simulink model "swps_2_xfer"  (Simulink 7.0)
settings: Solver=ode23s  StartTime=0.0  StopTime=inf  MaxStep=.02/50e3  RelTol=1e-3
values from neighbouring files (symbols this model uses):
  a = [1 5726094.8537 1.28575913301e+14 5.9794238322e+20 5.92198785204e+27 2.12389820757e+34 1.13681638083e+41 2.81062253129e+47 7.3943533776e+53 8.72896491872e+59]    [lpf_coefs.mat]
  b = [0 36927.0233589 -2.57790101622e-05 1.2013848239e+19 -1092387632.02 1.28157428918e+33 2.40587360249e+23 5.61084731217e+46 9.8548958414e+36 8.72896491872e+59]    [lpf_coefs.mat]
undefined symbols (not defined in the file or in its folder): c, d, dfilt, gcbh, magnitude, powericon
libraries: powerlib x9, dspindex x8, dspsigops x4, dspbuff3 x3, dspxfrm3 x3, dsparch4 x2, dspsnks4 x2, dspsrcs4 x1, dspmtrx3 x1, simulink x1, simulink_extras x1
CloseFcn:
  | rtwprivate ssgencode ModelCloseRequest swps_2
settings Model: Creator=dbenson  LastModifiedBy=Owner
settings SolverCC: InitialStep=.01/50e3  ZeroCrossControl=EnableAll
settings DataIOCC: LimitDataPoints=off  SaveOutput=off  SignalLogging=off  SaveTime=off  SignalLoggingName=sigsOut
settings OptimizationCC: BooleanDataType=off  OptimizeModelRefInitCode=on  LifeSpan=1
settings DebuggingCC: SaveWithParameterizedLinksMsg=none  SignalResolutionControl=TryResolveAllWithWarning  SolverPrmCheckMsg=none  MultiTaskDSMMsg=warning  MultiTaskCondExecSysMsg=none  StrictBusMsg=None
settings RTWCC: SystemTargetFile=ert.tlc  TemplateMakefile=ert_default_tmf  Description=Real-Time Workshop Embedded Coder (no auto configuration)  GenerateReport=on  ProcessScript=ert_make_rtw_hook  IncludeHyperlinkInReport=on  LaunchReport=on  IncludeERTFirstTime=on
settings CodeAppCC: IgnoreCustomStorageClasses=off
settings ERTTargetCC: TargetFcnLib=ansi_tfl_tmw.mat  GenFloatMathFcnCalls=ANSI_C  GenerateSampleERTMain=on  GenerateErtSFunction=on  InlinedParameterPlacement=NonHierarchical  ERTCustomFileTemplate=example_file_process.tlc

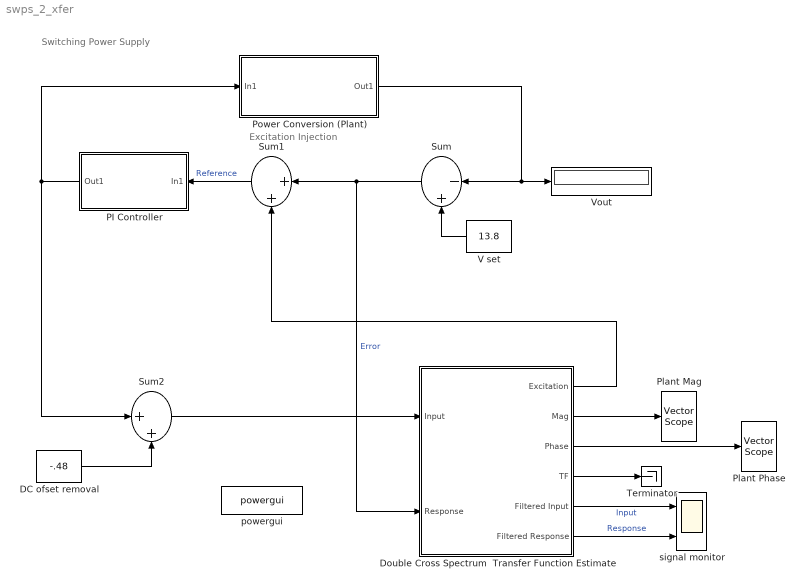
== system swps_2_xfer ==
  note: Switching Power Supply
  note: Excitation Injection
  DC ofset removal : Constant  Value=-.48  OutDataType=sfix(16)  OutScaling=2^0
  Double Cross Spectrum  Transfer Function Estimate : Subsystem  Description=Spectrum Analyzer  mask{BW=5e3, NFFT=128, Level=.02, Chirp=off, Avg_fac=10, Nholdoff=2, Unwrap=off}
      mask prompts: BW "Bandwidth (Hz)"; NFFT "FFT Length (power of 2)"; Level "Excitation Level"; Chirp "Chirp Excitation"; Avg_fac "Averaging Factor (>=1)"; Nholdoff "Hold Off  (in Frames)"; Unwrap "Unwrap Phase"
  PI Controller : Subsystem  Orientation=left
  Plant Mag : dspsnks4/Vector Scope  DialogController=dspdialog.VectorScope  DialogControllerArgs=DataTag9  ScopeProperties=on  Domain=Frequency  HorizSpan=1  DisplayProperties=off  AxisGrid=on  Memory=off  FrameNumber=on  AxisLegend=off  AxisZoom=off  OpenScopeAtSimStart=on  OpenScopeImmediately=off  FigPos=[7 35 334 255]  AxisProperties=off  XUnits=Hertz  XRange=[0...Fs/2]  InheritXIncr=on  XIncr=1  XLabel=Time  XLimit=Auto  XMin=0  XMax=1  XStart=0  YUnits=dB  YLabel=Amplitude  LineProperties=off
      settings: YMin=-30  YMax=30
  Plant Phase : dspsnks4/Vector Scope  DialogController=dspdialog.VectorScope  DialogControllerArgs=DataTag10  ScopeProperties=on  Domain=Frequency  HorizSpan=1  DisplayProperties=off  AxisGrid=on  Memory=off  FrameNumber=on  AxisLegend=off  AxisZoom=off  OpenScopeAtSimStart=on  OpenScopeImmediately=off  FigPos=[350 28 337 266]  AxisProperties=off  XUnits=Hertz  XRange=[0...Fs/2]  InheritXIncr=on  XIncr=1  XLabel=Time  XLimit=Auto  XMin=0  XMax=1  XStart=0  YUnits=Magnitude  YLabel=Phase  LineProperties=off
      settings: YMin=-50  YMax=200
  Power Conversion (Plant) : Subsystem
  Sum : Sum  Orientation=left  Inputs=|-+  OutDataType=sfix(16)  OutScaling=2^0  SaturateOnIntegerOverflow=on  InputSameDT=on
  Sum1 : Sum  Orientation=left  Inputs=|++  OutDataType=sfix(16)  OutScaling=2^0  SaturateOnIntegerOverflow=on  InputSameDT=on
  Sum2 : Sum  Inputs=|++  OutDataType=sfix(16)  OutScaling=2^0  SaturateOnIntegerOverflow=on  InputSameDT=on
  Terminator : Terminator
  "V set " : Constant  Orientation=left  Value=13.8  OutDataType=sfix(16)  OutScaling=2^0
  Vout : Display
      settings: Decimation=20
  powergui : powerlib/powergui  SystemSampleTime=-1  SimulationMode=Continuous  SampleTime=0  echomessages=off  RestoreLinks=warning  x0status=blocks  Frange=[0:2:500]  Ylog=off  Xlog=on  ShowGrid=off  save=off  variable=ZData  ZoomFFT=on  StartTime=0.0  cycles=1  DisplayStyle=1  fundamental=60  FreqAxis=off  MaxFrequency=1000  frequencyindice=0  frequencyindicesteady=1  RmsSteady=1  display=off  Ts=0  frequency=60  methode=off  HookPort=off  Interpol=off  SPID=off  FunctionMessages=off
  signal monitor : Scope  NumInputPorts=2
      settings: TimeRange=0.01  YMin=-0.75~-0.3  YMax=0.75~0.25  SaveName=ScopeData2
  wires:
  "V set "/1 -> Sum/2
  Power Conversion (Plant)/1(Out1) -> Sum/1, Vout/1
  PI Controller/1(Out1) -> Power Conversion (Plant)/1(In1), Sum2/1
  Sum/1 -> Sum1/1, Double Cross Spectrum  Transfer Function Estimate/2(Response)  "Error"
  Sum1/1 -> PI Controller/1(In1)  "Reference"
  Double Cross Spectrum  Transfer Function Estimate/2(Mag) -> Plant Mag/1
  Double Cross Spectrum  Transfer Function Estimate/3(Phase) -> Plant Phase/1
  Double Cross Spectrum  Transfer Function Estimate/1(Excitation) -> Sum1/2
  DC ofset removal/1 -> Sum2/2
  Double Cross Spectrum  Transfer Function Estimate/4(TF) -> Terminator/1
  Sum2/1 -> Double Cross Spectrum  Transfer Function Estimate/1(Input)
  Double Cross Spectrum  Transfer Function Estimate/5(Filtered Input) -> signal monitor/1  "Input"
  Double Cross Spectrum  Transfer Function Estimate/6(Filtered Response) -> signal monitor/2  "Response"

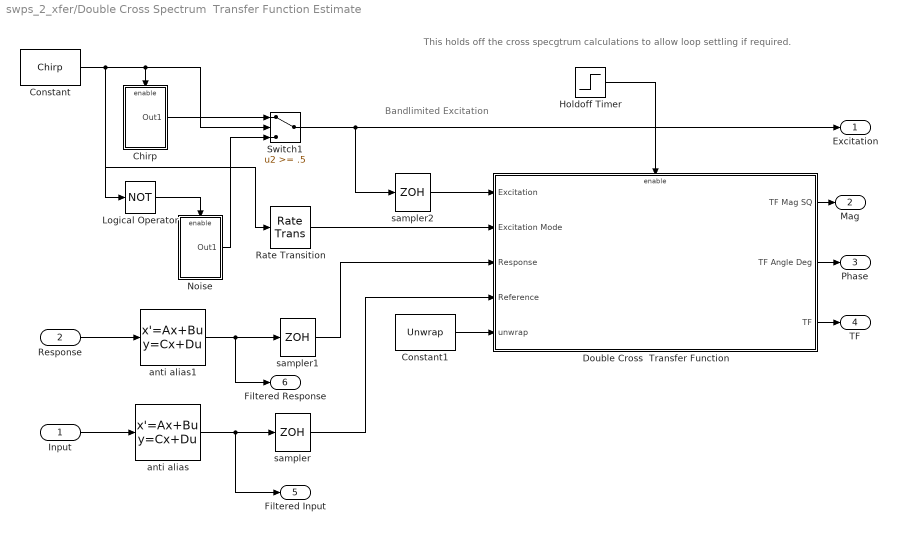
== system swps_2_xfer/Double Cross Spectrum  Transfer Function Estimate ==
  note: This holds off the cross specgtrum calculations
      |  to allow loop settling if required.
  note: Bandlimited Excitation
  Input : Inport  OutDataType=sfix(16)  OutScaling=2^0
  Response : Inport  Port=2  OutDataType=sfix(16)  OutScaling=2^0
  Chirp : Subsystem
  Constant : Constant  Value=Chirp  OutDataType=sfix(16)  OutScaling=2^0
  Constant1 : Constant  Value=Unwrap  OutDataType=sfix(16)  OutScaling=2^0
  "Double Cross  Transfer Function " : Subsystem  mask{NFFT=NFFT, Navg=Avg_fac, pcnt=100/1.28, BW=BW}
      mask prompts: NFFT "FFT length (power of 2):"; Navg "Spectral Averaging Factor (>=1):"; pcnt "Percentage of  Alias Free Data  (<=100)"; BW "Bandwidth"
      mask Display: disp('Double Cross\n Transfer Function \n Estimation (v1.0) ')
  Holdoff Timer : Step  Time=Nholdoff*NFFT/(2.56*BW)  SampleTime=1/(2.56*BW)
  Logical Operator : Logic  Operator=NOT  AllPortsSameDT=off  OutDataTypeMode=boolean
  Noise : Subsystem
  Rate Transition : RateTransition
  Switch1 : Switch  Threshold=.5
  anti alias : StateSpace  AncestorBlock=dsparch3/Analog Filter Design  A=a  B=b  C=c  D=d  mask(Analog Filter Design){method=Elliptic, filttype=Lowpass, N=8, Wlo=BW*2*pi, Whi=80, Rp=2, Rs=100}
      mask prompts: method "Design method:"; filttype "Filter type:"; N "Filter order:"; Wlo "Passband edge frequency (rad/s):"; Whi "(unused)"; Rp "Passband ripple in dB:"; Rs "Stopband attenuation in dB:"
      mask help: Design one of several standard analog filters, implemented in state-space form.
      mask init:
      | [a,b,c,d,h,w,str]=dspblkanalog('design', method,filttype,N,Wlo,Whi,Rp,Rs);
      mask Help: web(dspbhelp);
      mask StyleString: popup(Butterworth|Chebyshev I|Chebyshev II|Elliptic|Bessel),popup(Lowpass|Highpass|Bandpass|Bandstop),edit,edit,edit,edit,edit
      mask CallbackString: dspblkanalog|dspblkanalog|||||
      mask Display: plot(w,h); text(.05,.9,str);
  anti alias1 : StateSpace  AncestorBlock=dsparch3/Analog Filter Design  A=a  B=b  C=c  D=d  mask(Analog Filter Design){method=Elliptic, filttype=Lowpass, N=8, Wlo=BW*2*pi, Whi=80, Rp=2, Rs=100}
      mask prompts: method "Design method:"; filttype "Filter type:"; N "Filter order:"; Wlo "Passband edge frequency (rad/s):"; Whi "(unused)"; Rp "Passband ripple in dB:"; Rs "Stopband attenuation in dB:"
      mask help: Design one of several standard analog filters, implemented in state-space form.
      mask init:
      | [a,b,c,d,h,w,str]=dspblkanalog('design', method,filttype,N,Wlo,Whi,Rp,Rs);
      mask Help: web(dspbhelp);
      mask StyleString: popup(Butterworth|Chebyshev I|Chebyshev II|Elliptic|Bessel),popup(Lowpass|Highpass|Bandpass|Bandstop),edit,edit,edit,edit,edit
      mask CallbackString: dspblkanalog|dspblkanalog|||||
      mask Display: plot(w,h); text(.05,.9,str);
  sampler : ZeroOrderHold  SampleTime=1/(2.56*BW)
  sampler1 : ZeroOrderHold  SampleTime=1/(2.56*BW)
  sampler2 : ZeroOrderHold  SampleTime=1/(2.56*BW)
  Excitation : Outport  OutDataType=sfix(16)  OutScaling=2^0
  Mag : Outport  Port=2  OutDataType=sfix(16)  OutScaling=2^0
  Phase : Outport  Port=3  OutDataType=sfix(16)  OutScaling=2^0
  TF : Outport  Port=4  OutDataType=sfix(16)  OutScaling=2^0
  Filtered Input : Outport  Port=5  OutDataType=sfix(16)  OutScaling=2^0
  Filtered Response : Outport  Port=6  OutDataType=sfix(16)  OutScaling=2^0
  wires:
  "Double Cross  Transfer Function "/3("TF ") -> TF/1
  sampler/1 -> "Double Cross  Transfer Function "/4(Reference)
  "Double Cross  Transfer Function "/1(TF Mag SQ) -> Mag/1
  "Double Cross  Transfer Function "/2(TF Angle Deg) -> Phase/1
  Holdoff Timer/1 -> "Double Cross  Transfer Function "/Enable
  anti alias/1 -> Filtered Input/1, sampler/1
  Input/1 -> anti alias/1
  anti alias1/1 -> sampler1/1, Filtered Response/1
  Response/1 -> anti alias1/1
  sampler1/1 -> "Double Cross  Transfer Function "/3(Response)
  Chirp/1(Out1) -> Switch1/1
  Noise/1(Out1) -> Switch1/3
  Switch1/1 -> Excitation/1, sampler2/1
  Constant/1 -> Logical Operator/1, Chirp/Enable, Switch1/2, Rate Transition/1
  Logical Operator/1 -> Noise/Enable
  Constant1/1 -> "Double Cross  Transfer Function "/5(unwrap)
  sampler2/1 -> "Double Cross  Transfer Function "/1(Excitation)
  Rate Transition/1 -> "Double Cross  Transfer Function "/2(Excitation Mode)

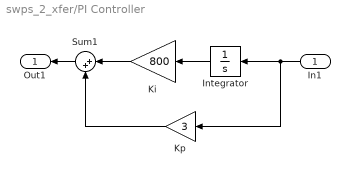
== system swps_2_xfer/PI Controller ==
  In1 : Inport  Orientation=left
  Integrator : Integrator  Orientation=left
  Ki : Gain  Orientation=left  Gain=800  ParameterDataType=sfix(16)  ParameterScaling=2^0  OutDataType=sfix(16)  OutScaling=2^0
  Kp : Gain  Orientation=left  Gain=3  ParameterDataType=sfix(16)  ParameterScaling=2^0  OutDataType=sfix(16)  OutScaling=2^0
  Sum1 : Sum  Orientation=left  Inputs=|++  OutDataType=sfix(16)  OutScaling=2^0  SaturateOnIntegerOverflow=on  InputSameDT=on
  Out1 : Outport  Orientation=left
  wires:
  In1/1 -> Kp/1, Integrator/1
  Integrator/1 -> Ki/1
  Kp/1 -> Sum1/2
  Sum1/1 -> Out1/1
  Ki/1 -> Sum1/1

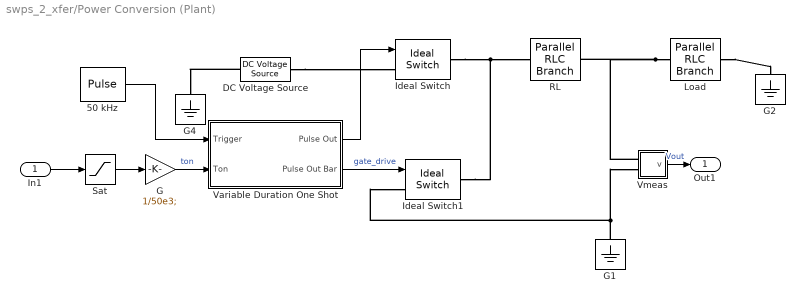
== system swps_2_xfer/Power Conversion (Plant) ==
  In1 : Inport
  50 kHz : DiscretePulseGenerator  PulseType=Time based  Period=1/50e3;  PulseWidth=50  PhaseDelay=1e-6
  DC Voltage Source : powerlib/Electrical Sources/DC Voltage Source  Description=source block  DialogController=POWERSYS.PowerSysDialog  SystemSampleTime=-1  Amplitude=30  Measurements=None
      settings: AttributesFormatString=\n
  G : Gain  Gain=1/50e3;  ParameterDataType=sfix(16)  ParameterScaling=2^0  OutDataType=sfix(16)  OutScaling=2^0  SaturateOnIntegerOverflow=on
  G1 : powerlib/Elements/Ground  Orientation=down  DialogController=POWERSYS.PowerSysDialog  PhysicalDomain=powersysdomain  SubClassName=unknown  LeftPortType=p1  RightPortType=p1  LConnTagsString=a
  G2 : powerlib/Elements/Ground  Orientation=down  DialogController=POWERSYS.PowerSysDialog  PhysicalDomain=powersysdomain  SubClassName=unknown  LeftPortType=p1  RightPortType=p1  LConnTagsString=a
  G4 : powerlib/Elements/Ground  Orientation=down  DialogController=POWERSYS.PowerSysDialog  PhysicalDomain=powersysdomain  SubClassName=unknown  LeftPortType=p1  RightPortType=p1  LConnTagsString=a
  Ideal Switch : powerlib/Power Electronics/Ideal Switch  DialogController=POWERSYS.PowerSysDialog  SystemSampleTime=-1  Ron=0.1  Lon=0  IC=0  Rs=0  Cs=0  Measurements=off
      settings: AttributesFormatString=\n
  Ideal Switch1 : powerlib/Power Electronics/Ideal Switch  DialogController=POWERSYS.PowerSysDialog  SystemSampleTime=-1  Ron=0.1  Lon=0  IC=0  Rs=0  Cs=0  Measurements=off
      settings: AttributesFormatString=\n
  Load : powerlib/Elements/Parallel RLC Branch  DialogController=POWERSYS.PowerSysDialog  PhysicalDomain=powersysdomain  SubClassName=unknown  LeftPortType=p1  RightPortType=p1  LConnTagsString=a  RConnTagsString=__new0  BranchType=RC  Resistance=2  Inductance=1.0  SetiL0=off  InitialCurrent=0  Capacitance=47e-6  Setx0=off  InitialVoltage=13.8  Measurements=None
  RL : powerlib/Elements/Parallel RLC Branch  DialogController=POWERSYS.PowerSysDialog  PhysicalDomain=powersysdomain  SubClassName=unknown  LeftPortType=p1  RightPortType=p1  LConnTagsString=a  RConnTagsString=__new0  BranchType=RL  Resistance=10000  Inductance=1e-3  SetiL0=off  InitialCurrent=0  Capacitance=1.0  Setx0=off  InitialVoltage=0  Measurements=None
  Sat : Saturate  UpperLimit=0.95  LowerLimit=.001
  Variable Duration One Shot : Subsystem
  Vmeas : Subsystem  Tag=PoWeRsYsTeMmEaSuReMeNt  AncestorBlock=powerlib/Measurements/Voltage Measurement  LoadFcn=powericon('psbloadfunction',gcbh,'Measurement Block','');  InitFcn=powericon('psbloadfunction',gcbh,'InitFcnOfSPSBlocks','Measurement Block');  mask(Voltage Measurement){PhasorSimulation=off, OutputType=Magnitude, PSBequivalent=0}
      mask prompts: PhasorSimulation "Phasor simulation"; OutputType "Output signal :"; PSBequivalent "Equivalent circuit"
      mask help: Ideal voltage measurement.
      mask init:
      | switch OutputType
      | case 1
      |     OutputSelection = 1;
      |     NormalMode = 2;
      |     PhasorMode = 1;
      | case 2
      |     OutputSelection =[2,3];
      |     NormalMode = 3;
      |     PhasorMode = [1,2];
      | case 3
      |     OutputSelection =[4,5];
      |     NormalMode = 3;
      |     PhasorMode = [1,2];
      | case 4
      |     OutputSelection =[4];
      |     NormalMode = 2;
      |     PhasorMode = 1;
      | end
      | %
      | if PhasorSimulation
      |     SelectionMode = PhasorMode;
      | else
      |     SelectionMode = NormalMode;
      | end
      settings: AttributesFormatString=\n  CopyFcn=powericon('psbloadfunction',gcbh,'Measurement Block','VerifyPhasor');  PreSaveFcn=powericon('psbloadfunction',gcbh,'ModelCloseFcn','');  CloseFcn=powericon('psbloadfunction',gcbh,'CloseFcn','');
      mask Help: web(psbhelp);
      mask StyleString: checkbox,popup(Complex|Real-Imag|Magnitude-Angle|Magnitude),edit
  Out1 : Outport
  wires:
  50 kHz/1 -> Variable Duration One Shot/1(Trigger)
  G/1 -> Variable Duration One Shot/2(Ton)  "ton"
  Sat/1 -> G/1
  Variable Duration One Shot/1(Pulse Out) -> Ideal Switch/1
  Variable Duration One Shot/2(Pulse Out Bar) -> Ideal Switch1/1  "gate_drive"
  In1/1 -> Sat/1
  Vmeas/1(v) -> Out1/1  "Vout"
  connections:
  DC Voltage Source/LConn1 -- G4/LConn1
  DC Voltage Source/RConn1 -- Ideal Switch/LConn1
  G1/LConn1 -- Vmeas/LConn2 -- Ideal Switch1/LConn1
  Load/RConn1 -- G2/LConn1
  Ideal Switch/RConn1 -- Ideal Switch1/RConn1 -- RL/LConn1
  Load/LConn1 -- RL/RConn1 -- Vmeas/LConn1

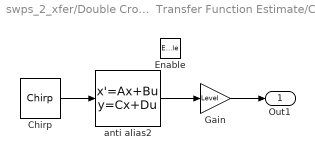
== system swps_2_xfer/Double Cross Spectrum  Transfer Function Estimate/Chirp ==
  Enable : EnablePort
  Chirp : dspsrcs4/Chirp  sweep=Linear  mode=Unidirectional  f0=0  f1=BW  t1=NFFT/(BW*2.56)  Tsweep=NFFT/(BW*2.56)  phase=3*pi/2  Ts=1/(2.56*BW)  spf=1  datatype=Double
  Gain : Gain  Gain=Level  ParameterDataType=sfix(16)  ParameterScaling=2^0  OutDataType=sfix(16)  OutScaling=2^0
  anti alias2 : StateSpace  AncestorBlock=dsparch3/Analog Filter Design  A=a  B=b  C=c  D=d  mask(Analog Filter Design){method=Elliptic, filttype=Lowpass, N=8, Wlo=BW*2*pi, Whi=80, Rp=2, Rs=100}
      mask prompts: method "Design method:"; filttype "Filter type:"; N "Filter order:"; Wlo "Passband edge frequency (rad/s):"; Whi "(unused)"; Rp "Passband ripple in dB:"; Rs "Stopband attenuation in dB:"
      mask help: Design one of several standard analog filters, implemented in state-space form.
      mask init:
      | [a,b,c,d,h,w,str]=dspblkanalog('design', method,filttype,N,Wlo,Whi,Rp,Rs);
      mask Help: web(dspbhelp);
      mask StyleString: popup(Butterworth|Chebyshev I|Chebyshev II|Elliptic|Bessel),popup(Lowpass|Highpass|Bandpass|Bandstop),edit,edit,edit,edit,edit
      mask CallbackString: dspblkanalog|dspblkanalog|||||
      mask Display: plot(w,h); text(.05,.9,str);
  Out1 : Outport
  wires:
  Chirp/1 -> anti alias2/1
  Gain/1 -> Out1/1
  anti alias2/1 -> Gain/1

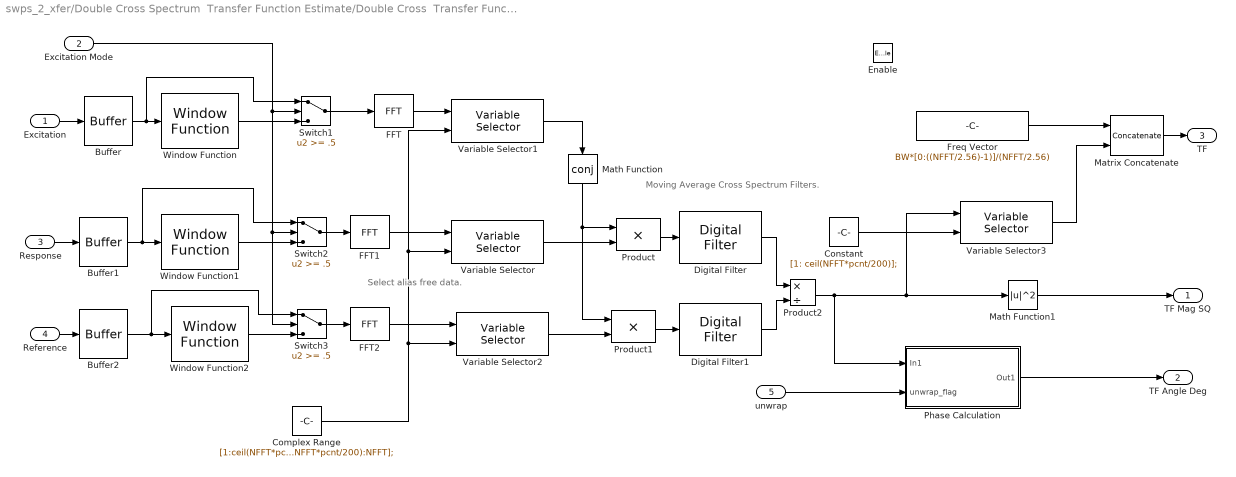
== system swps_2_xfer/Double Cross Spectrum  Transfer Function Estimate/Double Cross  Transfer Function  ==
  note: Moving Average Cross Spectrum Filters.
  note: Select alias free data.
  Excitation : Inport  OutDataType=sfix(16)  OutScaling=2^0
  Excitation Mode : Inport  Port=2  OutDataType=sfix(16)  OutScaling=2^0
  Response : Inport  Port=3  OutDataType=sfix(16)  OutScaling=2^0
  Reference : Inport  Port=4  OutDataType=sfix(16)  OutScaling=2^0
  unwrap : Inport  Port=5  OutDataType=sfix(16)  OutScaling=2^0
  Enable : EnablePort
  Buffer : dspbuff3/Buffer  N=NFFT  V=0  ic=0
  Buffer1 : dspbuff3/Buffer  N=NFFT  V=0  ic=0
  Buffer2 : dspbuff3/Buffer  N=NFFT  V=0  ic=0
  Complex Range : Constant  Value=[1:ceil(NFFT*pcnt/200),ceil(1+NFFT-NFFT*pcnt/200):NFFT];  OutDataType=sfix(16)  OutScaling=2^0
  Constant : Constant  Value=[1: ceil(NFFT*pcnt/200)];  OutDataType=sfix(16)  OutScaling=2^0
  Digital Filter : dsparch4/Digital Filter  DialogController=dspdialog.DigitalFilter  DialogControllerArgs=DataTag0  TypePopup=FIR (all zeros)  IIRFiltStruct=Direct form II transposed  AllPoleFiltStruct=Direct form  FIRFiltStruct=Direct form  CoeffSource=Specify via dialog  NumCoeffs=ones(1,Navg)  DenCoeffs=[1 0.1]  BiQuadCoeffs=[1 0.3 0.4 1 0.1 0.2]  LatticeCoeffs=[0.2 0.4]  denIgnore=on  FiltPerSampPopup=One filter per frame  IC=eps  ICnum=0  ICden=0  roundingMode=Floor  overflowMode=off  ScaleValues=1  scaleValueFracLength=14  stageInFracLength=15  stageOutFracLength=15  FilterSource=Specify via dialog  dfiltObjectName=dfilt.dffir([1 2 1])
  Digital Filter1 : dsparch4/Digital Filter  DialogController=dspdialog.DigitalFilter  DialogControllerArgs=DataTag1  TypePopup=FIR (all zeros)  IIRFiltStruct=Direct form II transposed  AllPoleFiltStruct=Direct form  FIRFiltStruct=Direct form  CoeffSource=Specify via dialog  NumCoeffs=ones(1,Navg)  DenCoeffs=[1 0.1]  BiQuadCoeffs=[1 0.3 0.4 1 0.1 0.2]  LatticeCoeffs=[0.2 0.4]  denIgnore=on  FiltPerSampPopup=One filter per frame  IC=eps  ICnum=0  ICden=0  roundingMode=Floor  overflowMode=off  ScaleValues=1  scaleValueFracLength=14  stageInFracLength=15  stageOutFracLength=15  FilterSource=Specify via dialog  dfiltObjectName=dfilt.dffir([1 2 1])
  FFT : dspxfrm3/FFT  DialogController=dspDDGCreate  DialogControllerArgs=DataTag2  CompMethod=Table lookup  TableOpt=Speed  BitRevOrder=off  InheritFFTLength=on  FFTLength=64  SkipNorm=off  firstCoeffMode=Specify word length  firstCoeffWordLength=16  firstCoeffFracLength=15  roundingMode=Floor  overflowMode=off
  FFT1 : dspxfrm3/FFT  DialogController=dspDDGCreate  DialogControllerArgs=DataTag3  CompMethod=Table lookup  TableOpt=Speed  BitRevOrder=off  InheritFFTLength=on  FFTLength=64  SkipNorm=off  firstCoeffMode=User-defined  firstCoeffWordLength=16  firstCoeffFracLength=15  roundingMode=Floor  overflowMode=off
  FFT2 : dspxfrm3/FFT  DialogController=dspDDGCreate  DialogControllerArgs=DataTag4  CompMethod=Table lookup  TableOpt=Speed  BitRevOrder=off  InheritFFTLength=on  FFTLength=64  SkipNorm=off  firstCoeffMode=User-defined  firstCoeffWordLength=16  firstCoeffFracLength=15  roundingMode=Floor  overflowMode=off
  Freq Vector : Constant  Value=BW*[0:((NFFT/2.56)-1)]/(NFFT/2.56)  OutDataType=sfix(16)  OutScaling=2^0
  Math Function : Math  Orientation=down  Operator=conj  OutDataType=sfix(16)  OutScaling=2^0  SaturateOnIntegerOverflow=on
  Math Function1 : Math  Operator=magnitude^2  OutDataType=sfix(16)  OutScaling=2^0  SaturateOnIntegerOverflow=on
  Matrix Concatenate : Concatenate  Mode=Multidimensional array  ConcatenateDimension=2
  Phase Calculation : Subsystem
  Product : Product  OutDataType=sfix(16)  OutScaling=2^0  SaturateOnIntegerOverflow=on  InputSameDT=on
  Product1 : Product  OutDataType=sfix(16)  OutScaling=2^0  SaturateOnIntegerOverflow=on  InputSameDT=on
  Product2 : Product  Inputs=*/  OutDataType=sfix(16)  OutScaling=2^0  SaturateOnIntegerOverflow=on  InputSameDT=on
  Switch1 : Switch  Threshold=.5
  Switch2 : Switch  Threshold=.5
  Switch3 : Switch  Threshold=.5
  Variable Selector{,1..3} (4 alike) : dspindex/Variable Selector  NumInputs=1  rowsOrCols=Rows  IdxMode=Variable  Elements=[1 3]  ZerOneIdxMode=One-based  errmode=Clip Index  FillMode=on  FillValues=0
  Window Function : dspsigops/Window Function  DialogController=dspDDGCreate  DialogControllerArgs=DataTag6  winmode=Apply window to input  wintype=Hann  sampmode=Continuous  samptime=1  N=64  Rs=50  beta=10  winsamp=Periodic  UserWindow=hamming  OptParams=off  UserParams={'symmetric'}  dataType=double  isSigned=on  wordLen=16  udDataType=sfix(16)  fracBitsMode=Best precision  numFracBits=15  roundingMode=Floor  overflowMode=off  numSidelobes=4  sidelobeLevel=-30
  Window Function1 : dspsigops/Window Function  DialogController=dspDDGCreate  DialogControllerArgs=DataTag7  winmode=Apply window to input  wintype=Hann  sampmode=Continuous  samptime=1  N=64  Rs=50  beta=10  winsamp=Periodic  UserWindow=hamming  OptParams=off  UserParams={'symmetric'}  dataType=double  isSigned=on  wordLen=16  udDataType=sfix(16)  fracBitsMode=Best precision  numFracBits=15  roundingMode=Floor  overflowMode=off  numSidelobes=4  sidelobeLevel=-30
  Window Function2 : dspsigops/Window Function  DialogController=dspDDGCreate  DialogControllerArgs=DataTag8  winmode=Apply window to input  wintype=Hann  sampmode=Continuous  samptime=1  N=64  Rs=50  beta=10  winsamp=Periodic  UserWindow=hamming  OptParams=off  UserParams={'symmetric'}  dataType=double  isSigned=on  wordLen=16  udDataType=sfix(16)  fracBitsMode=Best precision  numFracBits=15  roundingMode=Floor  overflowMode=off  numSidelobes=4  sidelobeLevel=-30
  TF Mag SQ : Outport  OutDataType=sfix(16)  OutScaling=2^0
  TF Angle Deg : Outport  Port=2  OutDataType=sfix(16)  OutScaling=2^0
  "TF " : Outport  Port=3  OutDataType=sfix(16)  OutScaling=2^0
  wires:
  Digital Filter1/1 -> Product2/2
  Product1/1 -> Digital Filter1/1
  Product/1 -> Digital Filter/1
  Digital Filter/1 -> Product2/1
  Variable Selector3/1 -> Matrix Concatenate/2
  Matrix Concatenate/1 -> "TF "/1
  Freq Vector/1 -> Matrix Concatenate/1
  Constant/1 -> Variable Selector3/2
  Variable Selector2/1 -> Product1/2
  FFT2/1 -> Variable Selector2/1
  Reference/1 -> Buffer2/1
  Buffer2/1 -> Window Function2/1, Switch3/1
  Complex Range/1 -> Variable Selector2/2, Variable Selector/2, Variable Selector1/2
  Phase Calculation/1(Out1) -> TF Angle Deg/1
  Response/1 -> Buffer1/1
  Excitation/1 -> Buffer/1
  FFT1/1 -> Variable Selector/1
  Math Function/1 -> Product1/1, Product/1
  FFT/1 -> Variable Selector1/1
  Math Function1/1 -> TF Mag SQ/1
  Buffer/1 -> Window Function/1, Switch1/1
  Buffer1/1 -> Window Function1/1, Switch2/1
  Product2/1 -> Phase Calculation/1(In1), Variable Selector3/1, Math Function1/1
  Variable Selector/1 -> Product/2
  Variable Selector1/1 -> Math Function/1
  Window Function/1 -> Switch1/3
  Switch1/1 -> FFT/1
  Window Function1/1 -> Switch2/3
  Switch2/1 -> FFT1/1
  Window Function2/1 -> Switch3/3
  Switch3/1 -> FFT2/1
  Excitation Mode/1 -> Switch1/2, Switch3/2, Switch2/2
  unwrap/1 -> Phase Calculation/2(unwrap_flag)

== system swps_2_xfer/Double Cross Spectrum  Transfer Function Estimate/Noise ==
  Enable : EnablePort
  Uniform Random Number : UniformRandomNumber  Minimum=-Level  Maximum=Level  SampleTime=1/(2.56*BW)
  anti alias2 : StateSpace  AncestorBlock=dsparch3/Analog Filter Design  A=a  B=b  C=c  D=d  mask(Analog Filter Design){method=Elliptic, filttype=Lowpass, N=8, Wlo=BW*2*pi, Whi=80, Rp=2, Rs=100}
      mask prompts: method "Design method:"; filttype "Filter type:"; N "Filter order:"; Wlo "Passband edge frequency (rad/s):"; Whi "(unused)"; Rp "Passband ripple in dB:"; Rs "Stopband attenuation in dB:"
      mask help: Design one of several standard analog filters, implemented in state-space form.
      mask init:
      | [a,b,c,d,h,w,str]=dspblkanalog('design', method,filttype,N,Wlo,Whi,Rp,Rs);
      mask Help: web(dspbhelp);
      mask StyleString: popup(Butterworth|Chebyshev I|Chebyshev II|Elliptic|Bessel),popup(Lowpass|Highpass|Bandpass|Bandstop),edit,edit,edit,edit,edit
      mask CallbackString: dspblkanalog|dspblkanalog|||||
      mask Display: plot(w,h); text(.05,.9,str);
  Out1 : Outport
  wires:
  Uniform Random Number/1 -> anti alias2/1
  anti alias2/1 -> Out1/1

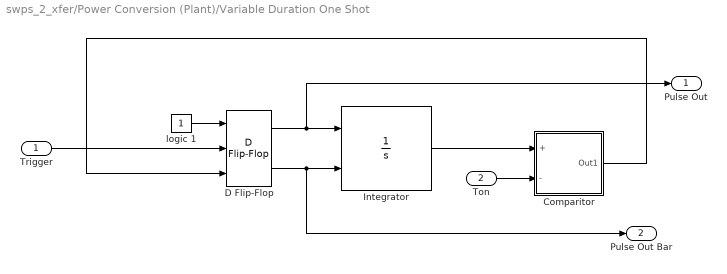
== system swps_2_xfer/Power Conversion (Plant)/Variable Duration One Shot ==
  Trigger : Inport  OutDataType=sfix(16)  OutScaling=2^0
  Ton : Inport  Port=2  OutDataType=sfix(16)  OutScaling=2^0
  Comparitor : Subsystem
  D Flip-Flop : simulink_extras/Flip Flops/D Flip-Flop  SystemSampleTime=-1
  Integrator : Integrator  ExternalReset=level
  logic 1 : Constant  OutDataType=sfix(16)  OutScaling=2^0
  Pulse Out : Outport  OutDataType=sfix(16)  OutScaling=2^0
  Pulse Out Bar : Outport  Port=2  OutDataType=sfix(16)  OutScaling=2^0
  wires:
  D Flip-Flop/2 -> Integrator/2, Pulse Out Bar/1
  logic 1/1 -> D Flip-Flop/1
  Integrator/1 -> Comparitor/1(+)
  D Flip-Flop/1 -> Integrator/1, Pulse Out/1
  Trigger/1 -> D Flip-Flop/2
  Ton/1 -> Comparitor/2(-)
  Comparitor/1(Out1) -> D Flip-Flop/3

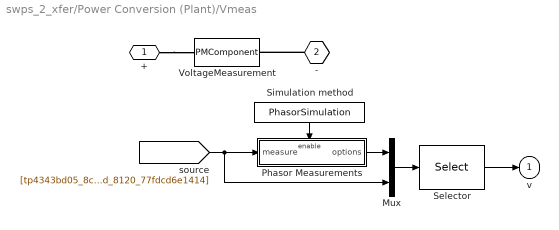
== system swps_2_xfer/Power Conversion (Plant)/Vmeas ==
  Mux : Mux  Inputs=2
  Phasor Measurements : Subsystem  TreatAsAtomicUnit=on
  Selector : Selector  InputPortWidth=length(OutputSelection)+1  IndexOptions=Index vector (dialog)  Indices=SelectionMode  OutputSizes=1
  Simulation method : Constant  Orientation=down  Value=PhasorSimulation  OutDataType=sfix(16)  OutScaling=2^0
  VoltageMeasurement : PMComponent  PhysicalDomain=powersysdomain  LeftPortType=p1  RightPortType=p1  LConnTagsString=+  RConnTagsString=-
      mask Type: InnerPowersysBlock
  + : PMIOPort  Port=1  Side=Left
  - : PMIOPort  Orientation=left  Port=2  Side=Left
  v : Outport  OutDataType=sfix(16)  OutScaling=2^0  InitialOutput=0
  wires:
  Simulation method/1 -> Phasor Measurements/Enable
  Mux/1 -> Selector/1
  Phasor Measurements/1(options) -> Mux/1
  Selector/1 -> v/1
  [tp4343bd05_8c15_42dd_8120_77fdcd6e1414] -> Phasor Measurements/1(measure), Mux/2
  connections:
  -/RConn1 -- VoltageMeasurement/RConn1
  +/RConn1 -- VoltageMeasurement/LConn1

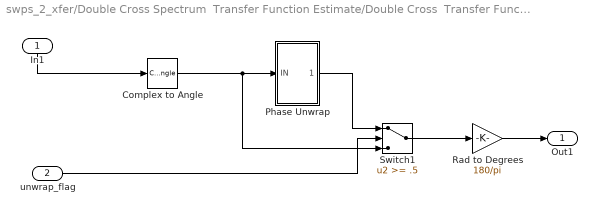
== system swps_2_xfer/Double Cross Spectrum  Transfer Function Estimate/Double Cross  Transfer Function /Phase Calculation ==
  In1 : Inport  Orientation=down
  unwrap_flag : Inport  Port=2  OutDataType=sfix(16)  OutScaling=2^0
  Complex to Angle : ComplexToMagnitudeAngle  Output=Angle
  Phase Unwrap : Subsystem
  Rad to Degrees : Gain  Gain=180/pi  ParameterDataType=sfix(16)  ParameterScaling=2^0  OutDataType=sfix(16)  OutScaling=2^0
  Switch1 : Switch  Threshold=.5
  Out1 : Outport
  wires:
  Rad to Degrees/1 -> Out1/1
  In1/1 -> Complex to Angle/1
  Complex to Angle/1 -> Switch1/3, Phase Unwrap/1(IN)
  Switch1/1 -> Rad to Degrees/1
  unwrap_flag/1 -> Switch1/2
  Phase Unwrap/1(Out1) -> Switch1/1

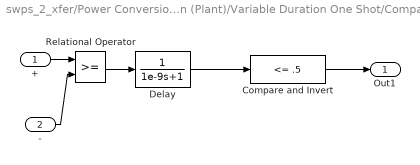
== system swps_2_xfer/Power Conversion (Plant)/Variable Duration One Shot/Comparitor ==
  + : Inport  OutDataType=sfix(16)  OutScaling=2^0
  - : Inport  Port=2  OutDataType=sfix(16)  OutScaling=2^0
  "Compare and Invert " : simulink/Logic and Bit Operations/Compare To Constant  SystemSampleTime=-1  relop=<=  const=.5  LogicOutDataTypeMode=uint8  ZeroCross=off
  Delay : TransferFcn  Denominator=[1e-9 1]
  Relational Operator : RelationalOperator  InputSameDT=on
  Out1 : Outport  OutDataType=sfix(16)  OutScaling=2^0
  wires:
  Relational Operator/1 -> Delay/1
  +/1 -> Relational Operator/1
  Delay/1 -> "Compare and Invert "/1
  -/1 -> Relational Operator/2
  "Compare and Invert "/1 -> Out1/1

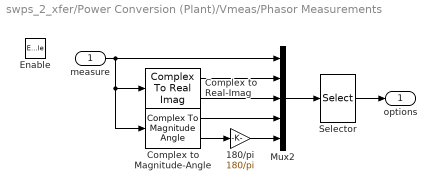
== system swps_2_xfer/Power Conversion (Plant)/Vmeas/Phasor Measurements ==
  measure : Inport  OutDataType=sfix(16)  OutScaling=2^0
  Enable : EnablePort
  180/pi : Gain  Gain=180/pi  ParameterDataType=sfix(16)  ParameterScaling=2^0  OutDataType=sfix(16)  OutScaling=2^0  SaturateOnIntegerOverflow=on
  Complex to Magnitude-Angle : ComplexToMagnitudeAngle
  Complex to Real-Imag : ComplexToRealImag
  Mux2 : Mux  Inputs=5
  Selector : Selector  InputPortWidth=5  IndexOptions=Index vector (dialog)  Indices=OutputSelection  OutputSizes=1
  options : Outport  OutDataType=sfix(16)  OutScaling=2^0  InitialOutput=0
  wires:
  Mux2/1 -> Selector/1
  measure/1 -> Complex to Magnitude-Angle/1, Complex to Real-Imag/1, Mux2/1
  Complex to Real-Imag/1 -> Mux2/2
  Complex to Real-Imag/2 -> Mux2/3
  Complex to Magnitude-Angle/1 -> Mux2/4
  Complex to Magnitude-Angle/2 -> 180/pi/1
  180/pi/1 -> Mux2/5
  Selector/1 -> options/1

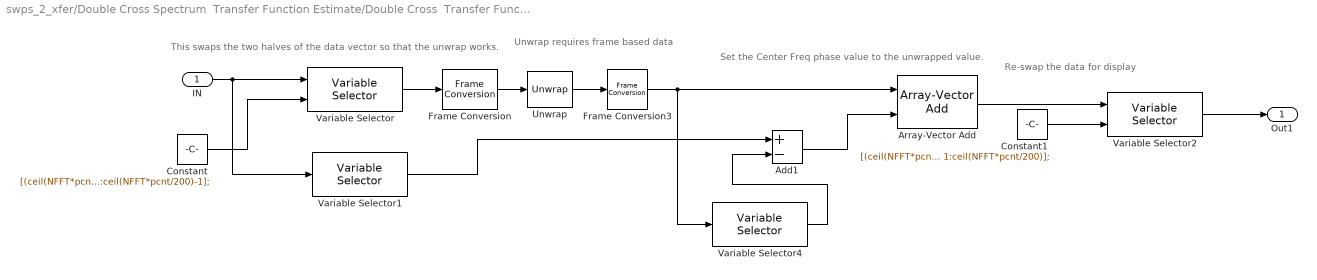
== system swps_2_xfer/Double Cross Spectrum  Transfer Function Estimate/Double Cross  Transfer Function /Phase Calculation/Phase Unwrap ==
  note: This swaps the two halves of the data vector
      | so that the unwrap works.
  note: Set the Center Freq phase value to the unwrapped value.
  note: Re-swap the data for display
  note: Unwrap requires frame based data
  IN : Inport  OutDataType=sfix(16)  OutScaling=2^0
  Add1 : Sum  Inputs=+-  OutDataType=sfix(16)  OutScaling=2^-10
  Array-Vector Add : dspmtrx3/Array-Vector Add  DialogController=dspDDGCreate  DialogControllerArgs=DataTag5  Dimension=2  V_Source=Input port  V_VectFromMask=[0.5 0.25]  roundingMode=Floor  overflowMode=off
  Constant : Constant  Value=[(ceil(NFFT*pcnt/200)):ceil(NFFT*pcnt/100) 1:ceil(NFFT*pcnt/200)-1];  OutDataType=sfix(16)  OutScaling=2^0
  Constant1 : Constant  Value=[(ceil(NFFT*pcnt/200)+1):ceil(NFFT*pcnt/100) 1:ceil(NFFT*pcnt/200)];  OutDataType=sfix(16)  OutScaling=2^0
  Frame Conversion : FrameConversion
  Frame Conversion3 : FrameConversion  OutFrame=Sample based
  Unwrap : dspsigops/Unwrap  running=on  tol=pi
  Variable Selector : dspindex/Variable Selector  NumInputs=1  rowsOrCols=Rows  IdxMode=Variable  Elements=[1 3]  ZerOneIdxMode=One-based  errmode=Clip Index  FillMode=on  FillValues=0
  Variable Selector1 : dspindex/Variable Selector  NumInputs=1  rowsOrCols=Rows  IdxMode=Fixed  Elements=[1]  ZerOneIdxMode=One-based  errmode=Clip Index  FillMode=on  FillValues=0
  Variable Selector2 : dspindex/Variable Selector  NumInputs=1  rowsOrCols=Rows  IdxMode=Variable  Elements=[1 3]  ZerOneIdxMode=One-based  errmode=Clip Index  FillMode=on  FillValues=0
  Variable Selector4 : dspindex/Variable Selector  NumInputs=1  rowsOrCols=Rows  IdxMode=Fixed  Elements=length([(ceil(NFFT*pcnt/200)+1):ceil(NFFT*pcnt/100) 1:ceil(NFFT*pcnt/200)] )/2+1  ZerOneIdxMode=One-based  errmode=Clip Index  FillMode=on  FillValues=0
  Out1 : Outport  OutDataType=sfix(16)  OutScaling=2^0
  wires:
  Frame Conversion/1 -> Unwrap/1
  Variable Selector2/1 -> Out1/1
  IN/1 -> Variable Selector/1, Variable Selector1/1
  Constant/1 -> Variable Selector/2
  Variable Selector/1 -> Frame Conversion/1
  Variable Selector1/1 -> Add1/1
  Unwrap/1 -> Frame Conversion3/1
  Variable Selector4/1 -> Add1/2
  Constant1/1 -> Variable Selector2/2
  Frame Conversion3/1 -> Variable Selector4/1, Array-Vector Add/1
  Add1/1 -> Array-Vector Add/2
  Array-Vector Add/1 -> Variable Selector2/1
